simulink library "tllib"  (R2021a)
settings: Solver=ode45  StartTime=0.0  StopTime=10.0  RelTol=1e-3  EnableMultiTasking=on
PostLoadFcn:
  | load_system('simulink')
undefined symbols (not defined in the file): DiscIntNeverNeededParam
libraries: simulink x6, $bdroot x3
(part 2 of 2)

== system tllib/AUTOSAR Blocks ==

== system tllib/Addfile ==
  dSPACE logo : Subsystem
      mask Display: image(ds_get_icon('dspace_logo_bg_white_l'))

== system tllib/Autodoc Customization ==
  dSPACE logo : Subsystem
      mask Display: image(ds_get_icon('dspace_logo_bg_white_l'))

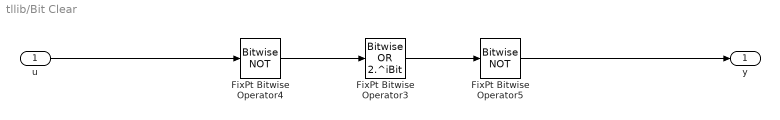
== system tllib/Bit Clear ==
  u : Inport
  FixPt Bitwise Operator3 : simulink/Logic and Bit Operations/Bitwise Operator  logicop=OR  UseBitMask=on  BitMask=2.^iBit  BitMaskRealWorld=Stored Integer
  FixPt Bitwise Operator4 : simulink/Logic and Bit Operations/Bitwise Operator  logicop=NOT  UseBitMask=off  BitMask=2.^iBit  BitMaskRealWorld=Stored Integer
  FixPt Bitwise Operator5 : simulink/Logic and Bit Operations/Bitwise Operator  logicop=NOT  UseBitMask=off  BitMask=2.^iBit  BitMaskRealWorld=Stored Integer
  y : Outport
  wires:
  FixPt Bitwise Operator5/1 -> y/1
  u/1 -> FixPt Bitwise Operator4/1
  FixPt Bitwise Operator4/1 -> FixPt Bitwise Operator3/1
  FixPt Bitwise Operator3/1 -> FixPt Bitwise Operator5/1

== system tllib/Bit Set ==
  u : Inport
  FixPt Bitwise Operator1 : simulink/Logic and Bit Operations/Bitwise Operator  logicop=OR  UseBitMask=on  BitMask=2.^iBit  BitMaskRealWorld=Stored Integer
  y : Outport
  wires:
  u/1 -> FixPt Bitwise Operator1/1
  FixPt Bitwise Operator1/1 -> y/1

== system tllib/Demos ==

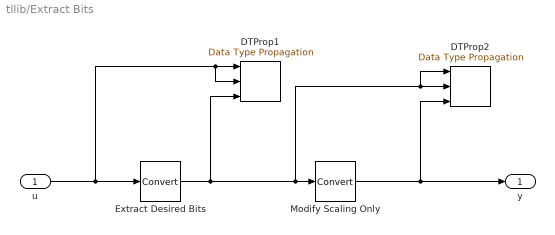
== system tllib/Extract Bits ==
  u : Inport
  DTProp1 : simulink/Signal Attributes/Data Type Propagation  PropDataType=fixdt(1, 16)  IfRefDouble=double  IfRefSingle=single  IsSigned=IsSigned1  NumBitsBase=NumBits1  NumBitsMult=0.5  NumBitsAdd=0  NumBitsAllowFinal=1:128  PropScaling=2^-10  ValuesUsedBestPrec=[5 -7]  SlopeBase=PosRange1  SlopeMult=2^0  SlopeAdd=0  BiasBase=Bias1  BiasMult=1  BiasAdd=0
      settings: SourceProductBaseCode=SL
  DTProp2 : simulink/Signal Attributes/Data Type Propagation  PropDataType=fixdt(1, 16)  IfRefDouble=double  IfRefSingle=single  IsSigned=IsSigned1  NumBitsBase=NumBits1  NumBitsMult=1  NumBitsAdd=0  NumBitsAllowFinal=1:128  PropScaling=1  ValuesUsedBestPrec=[5 -7]  SlopeBase=Slope1  SlopeMult=0  SlopeAdd=1  BiasBase=Bias1  BiasMult=0  BiasAdd=0
      settings: SourceProductBaseCode=SL
  Extract Desired Bits : DataTypeConversion  DisableCoverage=on
  Modify Scaling Only : DataTypeConversion  ConvertRealWorld=Stored Integer (SI)
  y : Outport
  wires:
  Modify Scaling Only/1 -> DTProp2/3, y/1
  u/1 -> Extract Desired Bits/1, DTProp1/2, DTProp1/1
  Extract Desired Bits/1 -> DTProp2/1, DTProp2/2, Modify Scaling Only/1, DTProp1/3

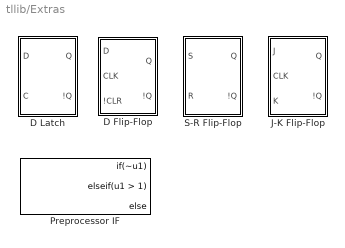
== system tllib/Extras ==
  D Flip-Flop : Subsystem  mask(TL_DFlipFlop){data={'date',730486}}
      mask help: SimulinkBlocks:simulink_extras:DFlipFlop_MD
      settings: CopyFcn=if exist('tl_reset_reviewflag','file')==2,tl_reset_reviewflag(gcbh);end  DeleteFcn=if exist('delete_tlblock','file')==2,delete_tlblock(gcbh);end  NameChangeFcn=if exist('rename_tlblock','file')==2,rename_tlblock(gcbh);end  OpenFcn=if exist('tl_open_blockdlg','file')==2,tl_open_blockdlg(gcbh);else,open_system(gcbh,'mask');end
      mask Help: eval(['if exist(''tl_online_help'',''file'') == 2, tl_online_help(''Topic'',''TL_DFlipFlop''),else, web([docroot ''/simulink/ref_extras/dflipflop.html'']),end'])
      mask Display: plot([-0.1, 1.05, NaN, -0.1, 1.05],[.01, .01, NaN, .99, .99]);
  D Latch : Subsystem  mask(TL_DLatch){data={'date',730486}}
      mask help: SimulinkBlocks:simulink_extras:DLatch_MD
      settings: CopyFcn=if exist('tl_reset_reviewflag') == 2, tl_reset_reviewflag(gcbh); end;  DeleteFcn=if exist('delete_tlblock','file')==2,delete_tlblock(gcbh);end  NameChangeFcn=if exist('rename_tlblock','file')==2,rename_tlblock(gcbh);end  OpenFcn=if exist('tl_open_blockdlg','file')==2,tl_open_blockdlg(gcbh);else,open_system(gcbh,'mask');end
      mask Help: eval(['if exist(''tl_online_help'',''file'') == 2, tl_online_help(''Topic'',''TL_DLatch''),else, web([docroot ''/simulink/ref_extras/dlatch.html'']),end'])
      mask Display: plot([-0.1, 1.05, NaN, -0.1, 1.05],[.01, .01, NaN, .99, .99]);
  J-K Flip-Flop : Subsystem  mask(TL_JKFlipFlop){initial_condition=0, data={'date',730486}}
      mask prompts: initial_condition "SimulinkBlocks:simulink_extras:InitialConditionstateOfQ_MP"
      mask help: SimulinkBlocks:simulink_extras:JKFlipFlop_MD
      settings: DeleteFcn=if exist('delete_tlblock','file')==2,delete_tlblock(gcbh);end  NameChangeFcn=if exist('rename_tlblock','file')==2,rename_tlblock(gcbh);end  OpenFcn=if exist('tl_open_blockdlg','file')==2,tl_open_blockdlg(gcbh);else,open_system(gcbh,'mask');end
      mask Help: eval(['if exist(''tl_online_help'',''file'') == 2, tl_online_help(''Topic'',''TL_JKFlipFlop''),else, web([docroot ''/simulink/ref_extras/jkflipflop.html'']),end'])
      mask Display: plot([-0.1, 1.05, NaN, -0.1, 1.05],[.01, .01, NaN, .99, .99]);
  Preprocessor IF : If  IfExpression=~u1  ElseIfExpressions=u1 > 1  mask(TL_PreProcessorIf){data={'date',730486}}
      settings: CopyFcn=if exist('tl_copyfcntllib', 'file') == 2, tl_copyfcntllib(gcbh); end;  DeleteFcn=if exist('delete_tlblock','file')==2,delete_tlblock(gcbh);end  NameChangeFcn=if exist('rename_tlblock','file')==2,rename_tlblock(gcbh);end  OpenFcn=if exist('tl_open_blockdlg','file')==2,tl_open_blockdlg(gcbh);else,open_system(gcbh,'parameter');end
      mask Help: eval(['if exist(''tl_online_help'',''file'') == 2, tl_online_help(''Topic'',''TL_PreProcessorIf''),else, web([''jar:file:///'',matlabroot,''/help/toolbox/simulink/help.jar!/slref/' lower(get_param(gcbh,'Blocktype')) '.html''], ''-helpbrowser''),end'])
      mask Display:
      | plot([-0.1, 1.05, NaN, -0.1, 1.05],[.01, .01, NaN, .99, .99]);
      | 
      | port_label('input', 1, 'u1')
      | port_label('output',1,'#if ~u1');
      | port_label('output',2,'#elif u1 > 1');
      | port_label('output',3,'#else');
  S-R Flip-Flop : Subsystem  mask(TL_SRFlipFlop){initial_condition=0, data={'date',730486}}
      mask prompts: initial_condition "SimulinkBlocks:simulink_extras:InitialConditionstateOfQ_MP"
      mask help: SimulinkBlocks:simulink_extras:SRFlipFlop_MD
      settings: DeleteFcn=if exist('delete_tlblock','file')==2,delete_tlblock(gcbh);end  NameChangeFcn=if exist('rename_tlblock','file')==2,rename_tlblock(gcbh);end  OpenFcn=if exist('tl_open_blockdlg','file')==2,tl_open_blockdlg(gcbh);else,open_system(gcbh,'mask');end
      mask Help: eval(['if exist(''tl_online_help'',''file'') == 2, tl_online_help(''Topic'',''TL_SRFlipFlop''),else, web([docroot ''/simulink/ref_extras/srflipflop.html'']),end'])
      mask Display: plot([-0.1, 1.05, NaN, -0.1, 1.05],[.01, .01, NaN, .99, .99]);

== system tllib/Function ==
  dSPACE logo : Subsystem
      mask Display: image(ds_get_icon('dspace_logo_bg_white_l'))

== system tllib/Help ==

== system tllib/RTOS blocks ==

== system tllib/Sample Blocks ==

== system tllib/Sink ==
  Inport : Inport  SampleTime=dt
  Terminator : Terminator
  wires:
  Inport/1 -> Terminator/1

== system tllib/Subsystem ==
  in. : Inport
  Subsystem : Subsystem  mask(TL_Enable){}
      settings: OpenFcn=warndlg(get_param(gcb,'MaskHelp'),'Serious Warning');
      mask Help: This subsystem keeps the TargetLink subsystem (subsystem with TargetLink blocks for production code generation), and is needed for the TargetLink simulation frame to work properly. DO NOT DELETE OR MODIFY IT!
  out. : Outport
  wires:
  in./1 -> Subsystem/1(in.)
  Subsystem/1(out.) -> out./1

== system tllib/Supported Simulink Blocks ==

== system tllib/TargetLink Main Dialog ==
  dSPACE logo : Subsystem
      mask Display: image(ds_get_icon('dspace_logo_bg_white_l'))

== system tllib/Tool Selector ==
  dSPACE logo : Subsystem
      mask Display: image(ds_get_icon('dspace_logo_bg_white_l'))

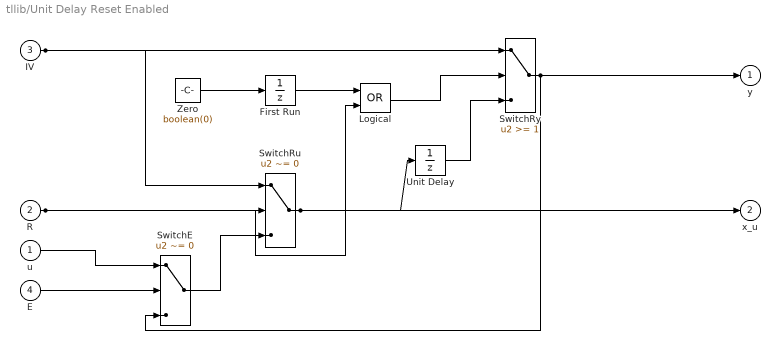
== system tllib/Unit Delay Reset Enabled ==
  u : Inport
  R : Inport  Port=2
  IV : Inport  Port=3
  E : Inport  Port=4
  First Run : UnitDelay  InitialCondition=useexternaliv  SampleTime=dt  HasFrameUpgradeWarning=on
  Logical : Logic  Operator=OR  AllPortsSameDT=off
  SwitchE : Switch  Criteria=u2 ~= 0  SaturateOnIntegerOverflow=on  InputSameDT=on
  SwitchRu : Switch  Criteria=u2 ~= 0  SaturateOnIntegerOverflow=on  InputSameDT=on
  SwitchRy : Switch  Threshold=1  SaturateOnIntegerOverflow=on  InputSameDT=on
  Unit Delay : UnitDelay  InitialCondition=X0  SampleTime=dt  HasFrameUpgradeWarning=on
  Zero : Constant  Value=boolean(0)
  y : Outport
  x_u : Outport  Port=2
  wires:
  IV/1 -> SwitchRy/1, SwitchRu/1
  Logical/1 -> SwitchRy/2
  Unit Delay/1 -> SwitchRy/3
  Zero/1 -> First Run/1
  First Run/1 -> Logical/1
  R/1 -> Logical/2, SwitchRu/2
  u/1 -> SwitchE/1
  E/1 -> SwitchE/2
  SwitchRy/1 -> SwitchE/3, y/1
  SwitchE/1 -> SwitchRu/3
  SwitchRu/1 -> Unit Delay/1, x_u/1

== system tllib/dSPACE logo ==

== system tllib/Addfile/dSPACE logo ==

== system tllib/Autodoc Customization/dSPACE logo ==

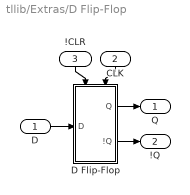
== system tllib/Extras/D Flip-Flop ==
  D : Inport
  CLK : Inport  Port=2
  !CLR : Inport  Port=3
  D Flip-Flop : Subsystem  TreatAsAtomicUnit=on
  Q : Outport  InitialOutput=0
  !Q : Outport  Port=2  InitialOutput=1
  wires:
  D Flip-Flop/2(!Q) -> !Q/1
  D/1 -> D Flip-Flop/1(D)
  D Flip-Flop/1(Q) -> Q/1
  !CLR/1 -> D Flip-Flop/Enable
  CLK/1 -> D Flip-Flop/Trigger

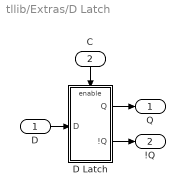
== system tllib/Extras/D Latch ==
  D : Inport
  C : Inport  Port=2
  D Latch : Subsystem  TreatAsAtomicUnit=on
  Q : Outport  InitialOutput=0
  !Q : Outport  Port=2  InitialOutput=1
  wires:
  C/1 -> D Latch/Enable
  D Latch/1(Q) -> Q/1
  D/1 -> D Latch/1(D)
  D Latch/2(!Q) -> !Q/1

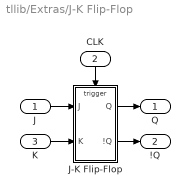
== system tllib/Extras/J-K Flip-Flop ==
  J : Inport
  CLK : Inport  Port=2
  K : Inport  Port=3
  J-K Flip-Flop : Subsystem  TreatAsAtomicUnit=on
  Q : Outport
  !Q : Outport  Port=2
  wires:
  CLK/1 -> J-K Flip-Flop/Trigger
  J-K Flip-Flop/1(Q) -> Q/1
  J/1 -> J-K Flip-Flop/1(J)
  K/1 -> J-K Flip-Flop/2(K)
  J-K Flip-Flop/2(!Q) -> !Q/1

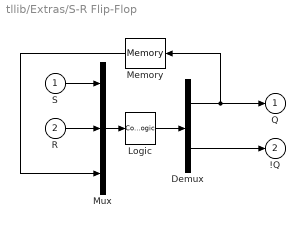
== system tllib/Extras/S-R Flip-Flop ==
  S : Inport
  R : Inport  Port=2
  Demux : Demux  Outputs=2
      settings: DisplayOption=none
  Logic : CombinatorialLogic  TruthTable=[0 1;1 0;0 1;0 1;1 0;1 0;0 0;0 0]
  Memory : Memory  InitialCondition=initial_condition  InheritSampleTime=on
  Mux : Mux  Inputs=3
  Q : Outport  InitialOutput=0
  !Q : Outport  Port=2  InitialOutput=1
  wires:
  Memory/1 -> Mux/3
  Mux/1 -> Logic/1
  Logic/1 -> Demux/1
  Demux/2 -> !Q/1
  Demux/1 -> Q/1, Memory/1
  S/1 -> Mux/1
  R/1 -> Mux/2

== system tllib/Function/dSPACE logo ==

== system tllib/Subsystem/Subsystem ==
  in. : Inport
  Subsystem : Subsystem  Tag=MIL Subsystem  mask(MIL Subsystem){}
      settings: CopyFcn=if exist('tl_copyfcn','file'), tl_copyfcn(gcbh); end  NameChangeFcn=if exist('tl_namechangefcn','file'), tl_namechangefcn(gcbh); end  DestroyFcn=if exist('update_tl_main_dlg','file'), update_tl_main_dlg('TL_subs_display'); end
  out. : Outport
  wires:
  in./1 -> Subsystem/1(InPort)
  Subsystem/1(OutPort) -> out./1

== system tllib/TargetLink Main Dialog/dSPACE logo ==

== system tllib/Tool Selector/dSPACE logo ==

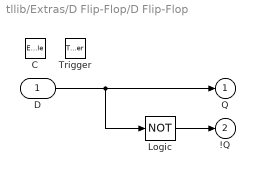
== system tllib/Extras/D Flip-Flop/D Flip-Flop ==
  D : Inport  LatchByDelayingOutsideSignal=on
  C : EnablePort
  Trigger : TriggerPort  VariantControl=(inherit)  StatesWhenEnabling=reset
  Logic : Logic  Operator=NOT  Inputs=1
  Q : Outport  OutputWhenDisabled=reset  InitialOutput=0
  !Q : Outport  Port=2  OutputWhenDisabled=reset  InitialOutput=1
  wires:
  D/1 -> Logic/1, Q/1
  Logic/1 -> !Q/1

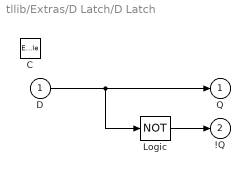
== system tllib/Extras/D Latch/D Latch ==
  D : Inport
  C : EnablePort
  Logic : Logic  Operator=NOT  Inputs=1
  Q : Outport  InitialOutput=0
  !Q : Outport  Port=2  InitialOutput=1
  wires:
  Logic/1 -> !Q/1
  D/1 -> Q/1, Logic/1

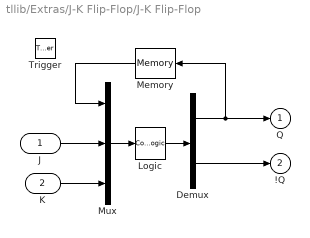
== system tllib/Extras/J-K Flip-Flop/J-K Flip-Flop ==
  J : Inport  LatchByDelayingOutsideSignal=on
  K : Inport  Port=2  LatchByDelayingOutsideSignal=on
  Trigger : TriggerPort  TriggerType=falling  VariantControl=(inherit)  StatesWhenEnabling=reset
  Demux : Demux  Outputs=2
      settings: DisplayOption=none
  Logic : CombinatorialLogic  TruthTable=[0 1; 0 1; 1 0; 1 0; 1 0; 0 1; 1 0; 0 1]
  Memory : Memory  InitialCondition=initial_condition  InheritSampleTime=on
  Mux : Mux  Inputs=3
  Q : Outport  InitialOutput=initial_condition
  !Q : Outport  Port=2  InitialOutput=~initial_condition
  wires:
  Mux/1 -> Logic/1
  Logic/1 -> Demux/1
  Demux/2 -> !Q/1
  Demux/1 -> Memory/1, Q/1
  Memory/1 -> Mux/1
  K/1 -> Mux/3
  J/1 -> Mux/2

== system tllib/Subsystem/Subsystem/Subsystem ==
  InPort : Inport  mask(TL_Inport){data={'date',730486}}
      settings: DeleteFcn=if exist('delete_tlblock','file')==2,delete_tlblock(gcbh);end  NameChangeFcn=if exist('rename_tlblock','file')==2,rename_tlblock(gcbh);end  OpenFcn=if exist('tl_open_blockdlg','file')==2,tl_open_blockdlg(gcbh);else,open_system(gcbh,'parameter');end
      settings: CopyFcn=|
      | if exist('tl_reset_reviewflag','file')==2
      |     tl_reset_reviewflag(gcbh);
      | end
      | if exist('tl_check_ports','file')
      |     tl_check_ports(gcbh);
      | end
      mask Help: eval(['if exist(''tl_online_help'',''file'') == 2, tl_online_help(''Topic'',''TL_Inport''),else, web([''jar:file:///'',matlabroot,''/help/toolbox/simulink/help.jar!/slref/' lower(get_param(gcbh,'Blocktype')) '.html''], ''-helpbrowser''),end'])
      mask Display: plot([0.2 0.35 NaN 0.65 0.8],[0 1 NaN 0 1]);
  OutPort : Outport  mask(TL_Outport){data={'date',730486}}
      settings: DeleteFcn=if exist('delete_tlblock','file')==2,delete_tlblock(gcbh);end  NameChangeFcn=if exist('rename_tlblock','file')==2,rename_tlblock(gcbh);end  OpenFcn=if exist('tl_open_blockdlg','file')==2,tl_open_blockdlg(gcbh);else,open_system(gcbh,'parameter');end
      settings: CopyFcn=|
      | if exist('tl_reset_reviewflag','file')==2
      |     tl_reset_reviewflag(gcbh);
      | end
      | if exist('tl_check_ports','file')
      |     tl_check_ports(gcbh);
      | end
      mask Help: eval(['if exist(''tl_online_help'',''file'') == 2, tl_online_help(''Topic'',''TL_Outport''),else, web([''jar:file:///'',matlabroot,''/help/toolbox/simulink/help.jar!/slref/' lower(get_param(gcbh,'Blocktype')) '.html''], ''-helpbrowser''),end'])
      mask Display: plot([0.2 0.35 NaN 0.65 0.8],[0 1 NaN 0 1]);
